simulink subsystem "Plant_Model_HT_Cooling_InnerLoop"  (R2022b)
settings: Solver=VariableStepAuto  StartTime=0.0  StopTime=10.0  RelTol=1e-3
values from neighbouring files (symbols this model uses):
  air_cp = 1004    [All_Properties.mat]    (also in cathode_subsystem_parameters.m; thermal_subsystem_parameters.m)
  air_HC_min = 10    [All_Properties.mat]    (also in cathode_subsystem_parameters.m; thermal_subsystem_parameters.m)
  air_HC_nom = 100    [All_Properties.mat]    (also in cathode_subsystem_parameters.m; thermal_subsystem_parameters.m)
  air_rho = 1.2    [All_Properties.mat]    (also in cathode_subsystem_parameters.m; thermal_subsystem_parameters.m)
  air_vel_nom = 1    [All_Properties.mat]    (also in cathode_subsystem_parameters.m; thermal_subsystem_parameters.m)
  coolant_initial_pressure = 0.111325    [All_Properties.mat]    (also in cathode_subsystem_parameters.m; thermal_subsystem_parameters.m)
  coolant_initial_temperature = 313.15    [All_Properties.mat]    (also in cathode_subsystem_parameters.m = 293.15; thermal_subsystem_parameters.m = 293.15)
  coolant_num_layers = 20    [All_Properties.mat]    (also in Plant_Model_HT_Cooling_Parameters.m; cathode_subsystem_parameters.m = 15; environment_parameters.m; stack_model_harness_parameters.m)
  coolant_num_passes = 12    [All_Properties.mat]    (also in Plant_Model_HT_Cooling_Parameters.m; cathode_subsystem_parameters.m = 20; environment_parameters.m; stack_model_harness_parameters.m)
  coolant_tube_D = 0.05    [All_Properties.mat]    (also in Plant_Model_HT_Cooling_Parameters.m; cathode_subsystem_parameters.m; environment_parameters.m; stack_model_harness_parameters.m)
  coolant_w_channels = 1    [All_Properties.mat]    (also in Plant_Model_HT_Cooling_Parameters.m; cathode_subsystem_parameters.m; environment_parameters.m; stack_model_harness_parameters.m)
  radiator_area_air = 0.1026    [All_Properties.mat]    (also in cathode_subsystem_parameters.m; thermal_subsystem_parameters.m)
  radiator_area_fins = 2.543625    [All_Properties.mat]    (also in cathode_subsystem_parameters.m; thermal_subsystem_parameters.m)
  radiator_area_primary = 0.444525    [All_Properties.mat]    (also in cathode_subsystem_parameters.m; thermal_subsystem_parameters.m = 2 * radiator_tube_length * radiator_width * (radiator_fin_ro)
  radiator_n_tubes = 20    [All_Properties.mat]    (also in cathode_subsystem_parameters.m; thermal_subsystem_parameters.m)
  radiator_tube_height = 0.0015    [All_Properties.mat]    (also in cathode_subsystem_parameters.m; thermal_subsystem_parameters.m)
  radiator_tube_length = 0.45    [All_Properties.mat]    (also in cathode_subsystem_parameters.m; thermal_subsystem_parameters.m)
  radiator_width = 0.025    [All_Properties.mat]    (also in cathode_subsystem_parameters.m; thermal_subsystem_parameters.m)
  stack_area = 300    [All_Properties.mat]    (also in Plant_Model_HT_Cooling_Parameters.m = 280; cathode_subsystem_parameters.m = 280; stack_model_parameters.m = 280; stack_subsystem_parameters.m)
  tcp_time_constant = 2    [All_Properties.mat]    (also in Plant_Model_HT_Cooling_Parameters.m; cathode_subsystem_parameters.m; thermal_subsystem_parameters.m)
  tcv_orifice_diameter = 0.045    [All_Properties.mat]    (also in Plant_Model_HT_Cooling_Parameters.m; cathode_subsystem_parameters.m; thermal_subsystem_parameters.m)
  tcv_time_constant = 0.2    [All_Properties.mat]    (also in Plant_Model_HT_Cooling_Parameters.m; cathode_subsystem_parameters.m; thermal_subsystem_parameters.m)
libraries: fl_lib x50, nesl_utility x40, SimscapeFluids_lib x7, eeGeneralControl x1
settings Model: Creator=stefan.notter  LastModifiedBy=stefan.notter

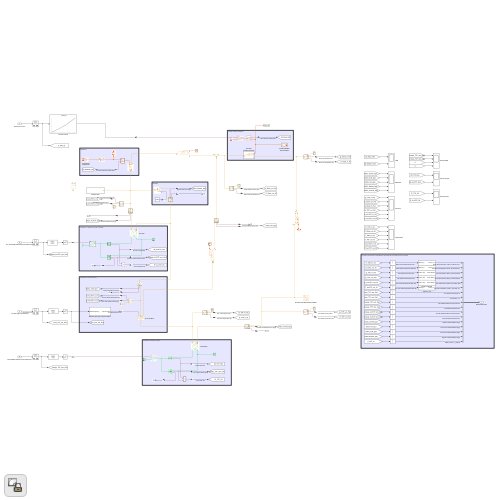
[thumbnail: Simulink's stored preview of the top-level diagram]
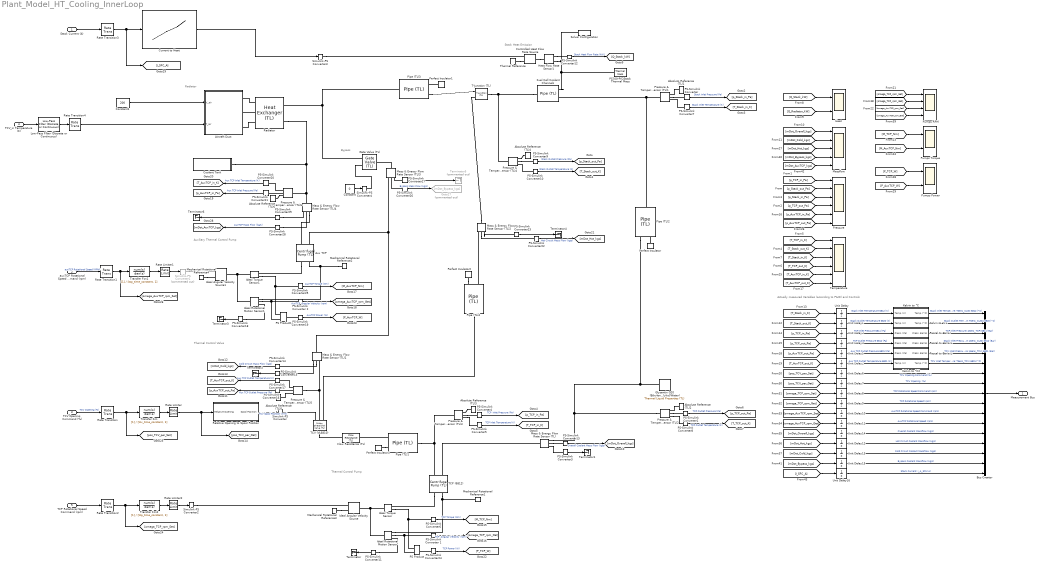
== system Plant_Model_HT_Cooling_InnerLoop ==
  note: Bypass
  note: Thermal Control Valve
  note: Actually measured Variables (according to P&ID) and Controls
  note: Stack Heat Emission
  note: Thermal Control Pump
  note: Radiator
  note: Auxiliary Thermal Control Pump
  Stack Current (A) : Inport
  auxTCP Rotational Speed Command (rpm) : Inport  Port=2
  TCV Opening Command (%) : Inport  Port=3
  TCV_in Temperature (K) : Inport  Port=4
  TCP Rotational Speed Command (rpm) : Inport  Port=5
  Absolute Reference (TL){1..6} (6 alike) : fl_lib/Thermal Liquid/Elements/Absolute Reference (TL)
  Aircraft Duct : Subsystem
  Aux TCP : SimscapeFluids_lib/Thermal Liquid/Pumps & Motors/Centrifugal Pump (TL)  pump_parameterization=fluids.thermal_liquid.pumps_motors.enum.CentrifugalPumpParameterization.Nominal  capacity_ref_nominal=6000/60 lpm  head_ref_nominal=|  power_ref_nominal=0.3 kW  head_ref_max=|  capacity_ref_max=12000/60 lpm  omega_ref_analytic=3500 rpm  flow_rate_1D_TLU=[1000, 2000, 3000, 4000, 5000, 6000, 7000, 8000, 9000, 1000] lpm  head_1D_TLU=[50, 47.5, 45, 40, 35, 25] m  power_1D_TLU=[.6, .75, .85, .93, .98, .99] kW  omega_ref_1D=3500 rpm  rho_ref_1D=998.21 kg/m^3  flow_rate_2D_TLU=[16.67, 23.33, 30, 40, 53.33, 60] lpm  omega_2D_TLU=[2450, 2800, 3150, 3500] rpm  head_2D_TLU=[25, 32.7, 42.5, 50; 24, 31.7, 41, 49; 22.7, 30.5, 39, 47.5; 20, 28, 36, 45; 15.7, 24, 32, 40; 12.5, 21, 29.5, 37.5] m  power_2D_TLU=[.28, .38, .5, .6; .31, .41, .55, .68; .33, .44, .6, .75; .36, .48, .65, .83; .38, .53, .72, .93; .39, .55, .75, .97] kW  rho_ref_2D=998.21 kg/m^3  diameter_ratio=1  mech_orientation=fluids.thermal_liquid.pumps_motors.enum.CentrifugalPumpMechOrientation.Positive  area=9.6211275016187417927918453612935e-4 m^2
      head_ref_nominal=|
      | 1.2*10^5/(1000*9.81)
      |  m
      head_ref_max=|
      | 1.55*10^5/(1000*9.81)
      |  m
      settings: InternalSimscapePortConfiguration="{\"Bottom\":[],\"Left\":[{\"id\":\"A\",\"label\":\"A\",\"type\":\"foundation.thermal_liquid.thermal_liquid\"},{\"id\":\"B\",\"label\":\"B\",\"type\":\"foundation.thermal_liquid.thermal_liquid\"}],\"Right\":[{\"id\":\"R\",\"label\":\"R\",\"type\":\"foundation.mechanical.rotational.rotational\"},{\"id\":\"C\",\"label\":\"C\",\"type\":\"foundation.mechanical.rotational.rotational\"}],\"Top\":[]}"
  Bus Creator : BusCreator  Inputs=17
  Constant : Constant  Value=0
  Constant1 : Constant  Value=200
  Controlled Heat Flow Rate Source : fl_lib/Thermal/Thermal Sources/Controlled Heat Flow Rate Source
  Coolant Tank : Subsystem  Tag=PublishSubsystem  mask(Coolant Tank){A=0.1, x_init=0.08}
      mask prompts: A "Tank area (m^2)"; x_init "Initial coolant level (m)"
      mask help: This subsystem models an expansion tank for the coolant system.
  Current to Heat : Lookup_n-D  NumberOfTableDimensions=1  BreakpointsForDimension1=[0:50:400]  Table=[0, 9932, 21438, 33442,47123, 59491, 77033, 93585, 112042]  InternalRulePriority=Speed  RndMeth=Simplest
  Flow Resistance (TL) : fl_lib/Thermal Liquid/Elements/Flow Resistance (TL)  delta_p_nominal=0.05 bar  mdot_nominal=1 kg/s  area=pi*tcv_orifice_diameter^2/4 m^2  laminar_fraction=1e-3
  Fuel Cell Coolant Channels : fl_lib/Thermal Liquid/Elements/Pipe (TL)  length=sqrt(stack_area) * coolant_num_passes cm  area=coolant_w_channels^2 * coolant_num_layers cm^2  Dh=coolant_w_channels cm  length_add=10 cm  roughness=15e-5 m  Re_lam=2000  Re_tur=4000  shape_factor=64  Nu_lam=3.66  dynamic_compressibility=simscape.enum.onoff.on  inertia=simscape.enum.onoff.off  p0=coolant_initial_pressure MPa  T0=coolant_initial_temperature K  mdot0=0 kg/s
  Gate Valve (TL) : SimscapeFluids_lib/Thermal Liquid/Valves & Orifices/Flow Control Valves/Gate Valve (TL)  diam_orifice=0.01 m  S_min=0 m  area_leak=1e-12 m^2  smoothing_factor=0.01  area=0.01 m^2  Cd=0.7  Re_c=12
      settings: InternalSimscapePortConfiguration="{\"Bottom\":[],\"Left\":[{\"id\":\"A\",\"label\":\"A\",\"type\":\"foundation.thermal_liquid.thermal_liquid\"},{\"id\":\"S\",\"label\":\"S\",\"type\":\"input\"}],\"Right\":[{\"id\":\"B\",\"label\":\"B\",\"type\":\"foundation.thermal_liquid.thermal_liquid\"}],\"Top\":[]}"
  Glysantin G20 (Ethylenglykol/Water) : SimscapeFluids_lib/Thermal Liquid/Utilities/Thermal Liquid Properties (TL)  fluid_list=fluids.thermal_liquid.utilities.enum.thermal_liquid_fluid_list.ethylene_glycol  concentration_param_EG=fluids.thermal_liquid.utilities.enum.thermal_liquid_concentration.volume_fraction  concentration_param_PG=fluids.thermal_liquid.utilities.enum.thermal_liquid_concentration.volume_fraction  c_mass_SW=3.5e-3  c_mass_EG=0.1  c_mass_PG=0.1  c_mass_GL=0.1  c_vol_EG=0.5  c_vol_PG=0.1  beta_const_EG=2.1791 GPa  beta_const_PG=2.1791 GPa  beta_const_GL=2.1791 GPa  p_min_EG=0.01 MPa  p_min_PG=0.01 MPa  p_min_GL=0.01 MPa  p_max_EG=50 MPa  p_max_PG=50 MPa  p_max_GL=50 MPa  p_atm=coolant_initial_pressure MPa
  Goto27 : Goto  Commented=on  GotoTag=mDot_Bypass_kgs
  Heat : Scope  NumInputPorts=2
  Heat Flow Rate Sensor1 : fl_lib/Thermal/Thermal Sensors/Heat Flow Rate Sensor
  Ideal Angular Velocity Source : fl_lib/Mechanical/Mechanical Sources/Ideal Angular Velocity Source
  Ideal Angular Velocity Source1 : fl_lib/Mechanical/Mechanical Sources/Ideal Angular Velocity Source
  Ideal Rotational Motion Sensor : fl_lib/Mechanical/Mechanical Sensors/Ideal Rotational Motion Sensor  reference=foundation.enum.MeasurementReference.difference  acceleration_port=false  velocity_port=true  position_port=true  wrap_angle=false  offset=0 rad
  Ideal Rotational Motion Sensor1 : fl_lib/Mechanical/Mechanical Sensors/Ideal Rotational Motion Sensor  reference=foundation.enum.MeasurementReference.difference  acceleration_port=false  velocity_port=true  position_port=true  wrap_angle=false  offset=0 rad
  Ideal Torque Sensor : fl_lib/Mechanical/Mechanical Sensors/Ideal Torque Sensor
  Ideal Torque Sensor1 : fl_lib/Mechanical/Mechanical Sensors/Ideal Torque Sensor
  Kelvin to °C : Subsystem
  Kelvin to °C1 : Subsystem
  Kelvin to °C2 : Subsystem
  Low-Pass Filter (Discrete or Continuous) : eeGeneralControl/Low-Pass Filter (Discrete or Continuous)  K=1  T=1  B=inf  A=-inf  init_option=Inherited from block input  x0=0  Ts=-1
  Mass & Energy Flow Rate Sensor (TL){,1..4} (5 alike) : fl_lib/Thermal Liquid/Sensors/Mass & Energy Flow Rate Sensor (TL)
      settings: InternalSimscapePortConfiguration="{\"Bottom\":[],\"Left\":[{\"id\":\"A\",\"label\":\"A\",\"type\":\"foundation.thermal_liquid.thermal_liquid\"}],\"Right\":[{\"id\":\"B\",\"label\":\"B\",\"type\":\"foundation.thermal_liquid.thermal_liquid\"},{\"id\":\"M\",\"label\":\"M\",\"type\":\"output\"},{\"id\":\"PHI\",\"label\":\"Phi\",\"type\":\"output\"}],\"Top\":[]}"
  Massflow : Scope  NumInputPorts=5
  Mechanical Rotational Reference{1..4} (4 alike) : fl_lib/Mechanical/Rotational Elements/Mechanical Rotational Reference
  PS Product : fl_lib/Physical Signals/Functions/PS Product
  PS Product1 : fl_lib/Physical Signals/Functions/PS Product
  PS-Simulink Converter{,1,3..5,7..11,13..18,20..23,26..29} (24 alike) : nesl_utility/PS-Simulink Converter  PhysicalDomain=network_engine_domain  SubClassName=ps_output  LeftPortType=input  RightPortType=output  PseudoPeriodic=off  Frequencies=[]  VectorFormat=inherit  Unit=inherit  AffineConversion=off
  PS-Simulink Converter 1 : nesl_utility/PS-Simulink Converter  PhysicalDomain=network_engine_domain  SubClassName=ps_output  LeftPortType=input  RightPortType=output  PseudoPeriodic=off  Frequencies=[]  VectorFormat=1-D array  Unit=rpm  AffineConversion=off
  PS-Simulink Converter 2 : nesl_utility/PS-Simulink Converter  PhysicalDomain=network_engine_domain  SubClassName=ps_output  LeftPortType=input  RightPortType=output  PseudoPeriodic=off  Frequencies=[]  VectorFormat=1-D array  Unit=rpm  AffineConversion=off
  PS-Simulink Converter12 : nesl_utility/PS-Simulink Converter  PhysicalDomain=network_engine_domain  SubClassName=ps_output  LeftPortType=input  RightPortType=output  PseudoPeriodic=off  Frequencies=[]  VectorFormat=1-D array  Unit=kW  AffineConversion=off
  PS-Simulink Converter19 : nesl_utility/PS-Simulink Converter  PhysicalDomain=network_engine_domain  SubClassName=ps_output  LeftPortType=input  RightPortType=output  PseudoPeriodic=off  Frequencies=[]  VectorFormat=inherit  Unit=W  AffineConversion=off
  PS-Simulink Converter24 : nesl_utility/PS-Simulink Converter  PhysicalDomain=network_engine_domain  SubClassName=ps_output  LeftPortType=input  RightPortType=output  PseudoPeriodic=off  Frequencies=[]  VectorFormat=inherit  Unit=W  AffineConversion=off
  PS-Simulink Converter25 : nesl_utility/PS-Simulink Converter  PhysicalDomain=network_engine_domain  SubClassName=ps_output  LeftPortType=input  RightPortType=output  PseudoPeriodic=off  Frequencies=[]  VectorFormat=inherit  Unit=N*m  AffineConversion=off
  PS-Simulink Converter6 : nesl_utility/PS-Simulink Converter  PhysicalDomain=network_engine_domain  SubClassName=ps_output  LeftPortType=input  RightPortType=output  PseudoPeriodic=off  Frequencies=[]  VectorFormat=inherit  Unit=N*m  AffineConversion=off
  PS100-P02Stack Thermal Mass : fl_lib/Thermal/Thermal Elements/Thermal Mass  mass=stack_thermal_mass kg  sp_heat=stack_specific_heat J/kg/K  num_ports=foundation.enum.numPorts2.one  T_specify=on  T_priority=High  T=coolant_initial_temperature K  T_nominal_specify=off  T_nominal_unit=K  T_nominal_value=1  Q_specify=off  Q_priority=None  Q=20e3 W  Q_nominal_specify=off  Q_nominal_unit=W  Q_nominal_value=1
  Pascal to Bar(a) : Subsystem
  Pascal to Bar(a)1 : Subsystem
  Pascal to Bar(a)2 : Subsystem
  Perfect Insulator{,1..3} (4 alike) : fl_lib/Thermal/Thermal Elements/Perfect Insulator  T_specify=off  T_priority=None  T=293.15 K  T_nominal_specify=off  T_nominal_unit=K  T_nominal_value=1
  Pipe (TL)1 : fl_lib/Thermal Liquid/Elements/Pipe (TL)  length=0.5 m  area=pi*coolant_tube_D^2/4 m^2  Dh=pi*coolant_tube_D*0.9 m  length_add=0.5 m  roughness=15e-6 m  Re_lam=2000  Re_tur=4000  shape_factor=64  Nu_lam=3.66  dynamic_compressibility=simscape.enum.onoff.on  inertia=simscape.enum.onoff.off  p0=coolant_initial_pressure MPa  T0=coolant_initial_temperature K  mdot0=0 kg/s
  Pipe (TL)2 : fl_lib/Thermal Liquid/Elements/Pipe (TL)  length=0.5 m  area=pi*coolant_tube_D^2/4 m^2  Dh=pi*coolant_tube_D*0.9 m  length_add=1 m  roughness=15e-6 m  Re_lam=2000  Re_tur=4000  shape_factor=64  Nu_lam=3.66  dynamic_compressibility=simscape.enum.onoff.on  inertia=simscape.enum.onoff.off  p0=coolant_initial_pressure MPa  T0=coolant_initial_temperature K  mdot0=0 kg/s
  Pipe (TL)3 : fl_lib/Thermal Liquid/Elements/Pipe (TL)  length=1 m  area=pi*coolant_tube_D^2/4 m^2  Dh=pi*coolant_tube_D*0.9 m  length_add=1 m  roughness=15e-6 m  Re_lam=2000  Re_tur=4000  shape_factor=64  Nu_lam=3.66  dynamic_compressibility=simscape.enum.onoff.on  inertia=simscape.enum.onoff.off  p0=coolant_initial_pressure MPa  T0=coolant_initial_temperature K  mdot0=0 kg/s
  Pipe (TL)4 : fl_lib/Thermal Liquid/Elements/Pipe (TL)  length=0.5 m  area=pi*coolant_tube_D^2/4 m^2  Dh=pi*coolant_tube_D*0.9 m  length_add=1 m  roughness=15e-6 m  Re_lam=2000  Re_tur=4000  shape_factor=64  Nu_lam=3.66  dynamic_compressibility=simscape.enum.onoff.on  inertia=simscape.enum.onoff.off  p0=coolant_initial_pressure MPa  T0=coolant_initial_temperature K  mdot0=0 kg/s
  Pressure : Scope  NumInputPorts=6
  Pressure & Temperature Sensor (TL){1..6} (6 alike) : fl_lib/Thermal Liquid/Sensors/Pressure & Temperature Sensor (TL)
      settings: InternalSimscapePortConfiguration="{\"Bottom\":[],\"Left\":[{\"id\":\"A\",\"label\":\"A\",\"type\":\"foundation.thermal_liquid.thermal_liquid\"}],\"Right\":[{\"id\":\"B\",\"label\":\"B\",\"type\":\"foundation.thermal_liquid.thermal_liquid\"},{\"id\":\"P\",\"label\":\"P\",\"type\":\"output\"},{\"id\":\"T\",\"label\":\"T\",\"type\":\"output\"}],\"Top\":[]}"
  Pumps Power : Scope  NumInputPorts=2
  Pumps RPM : Scope  NumInputPorts=4
  Pumps Torque : Scope  NumInputPorts=2
  Radiator : SimscapeFluids_lib/Fluid Network Interfaces/Heat Exchangers/Heat Exchanger (TL)  hex_type=3  shell_num=1  cross_type=4  NTU_TLU=[0.5, 1.0, 2.0, 3.0, 4.0, 5.0]  CR_TLU=[0.0, 0.25, 0.5, 0.75, 1.0]  eff_TLU=[0.3, 0.3, 0.3, 0.3, 0.3; 0.6, 0.55, 0.5, 0.47, 0.43; 0.85, 0.76, 0.68, 0.61, 0.55; 0.94, 0.83, 0.72, 0.65, 0.58; 0.98, 0.86, 0.75, 0.66, 0.58; 0.99, 0.86, 0.75, 0.66, 0.58]  R_wall=0.014/(381*radiator_n_tubes*radiator_width*radiator_tube_length) K/W  min_flow_area_1=radiator_n_tubes*(radiator_width*radiator_tube_height) m^2  Dh_press_1=4*(radiator_width*radiator_tube_height)/(2 * (radiator_width+radiator_tube_height)) m  liquid_volume_1=radiator_n_tubes*(radiator_width*radiator_tube_height)*radiator_tube_length m^3  Re_lam_1=2000  Re_tur_1=4000  pressure_loss_spec_1=2  pressure_loss_coeff_1=15  length_press_1=radiator_tube_length m  length_add_1=0.1 m  roughness_1=15e-6 m  Re_friction_TLU_1=[400.0, 1000.0, 1500.0, 3000.0, 4000.0, 6000.0, 10000.0, 20000.0, 40000.0, 60000.0, 100000.0, 100000000.0]  friction_factor_TLU_1=[0.264, 0.112, 0.071, 0.0417, 0.0387, 0.0268, 0.025, 0.0232, 0.0226, 0.022, 0.0214, 0.0214]  shape_factor_1=64  Re_Euler_TLU_1=[50.0, 500.0, 1000.0, 2000.0]  Euler_TLU_1=[4.4505, 0.6864, 0.4791, 0.3755]  heat_transfer_spec_1=2  heat_transfer_area_1=radiator_n_tubes*2*(radiator_tube_length*radiator_width+radiator_tube_length*radiator_tube_height) m^2  heat_coeff_1=2000 W/(m^2 * K)  length_heat_1=radiator_tube_length cm  Nu_lam_1=3.66  Re_Colburn_TLU_1=[100.0, 150.0, 1000.0]  Colburn_factor_TLU_1=[0.019, 0.013, 0.002]  Re_Nu_TLU_1=[100.0, 150.0, 1000.0]  Pr_Nu_TLU_1=[1.0, 10.0]  Nu_TLU_1=[3.72, 4.21; 3.75, 4.44; 4.21, 7.15]  fouling_factor_1=0 m^2*K/W  min_heat_coeff_1=5 W/(m^2 * K)  heat_transfer_area_2=radiator_area_primary+radiator_area_fins m^2  fouling_factor_2=0 m^2*K/W  min_heat_coeff_2=0.01 W/(m^2 * K)  dynamic_compressibility_1=1  T0_1=coolant_initial_temperature K  p0_1=coolant_initial_pressure MPa  mdot1_TLU=[.1, .2] kg/s  mdot2_TLU=[.2, .3] kg/s  SD_TLU=[35, 35; 50, 50] kW/K  Q_check=1  mdot_dp_TLU_1=[.1, .2] kg/s  p_diff_TLU_1=[.003, .005] MPa  T_ref_in_1=293.15 K  p_ref_in_1=0.101325 MPa  mdot_threshold_1=1e-3 kg/s  area_1=0.01 m^2
      settings: InternalSimscapePortConfiguration="{\"Bottom\":[],\"Left\":[{\"id\":\"A1\",\"label\":\"A1\",\"type\":\"foundation.thermal_liquid.thermal_liquid\"},{\"id\":\"B1\",\"label\":\"B1\",\"type\":\"foundation.thermal_liquid.thermal_liquid\"}],\"Right\":[{\"id\":\"H2\",\"label\":\"H2\",\"type\":\"foundation.thermal.thermal\"},{\"id\":\"C2\",\"label\":\"C2\",\"type\":\"input\"},{\"id\":\"HC2\",\"label\":\"HC2\",\"type\":\"input\"}],\"Top\":[]}"
  Rate Limiter : RateLimiter  RisingSlewLimit=45  FallingSlewLimit=-45  SampleTimeMode=inherited
  Rate Limiter1 : RateLimiter  RisingSlewLimit=1000  FallingSlewLimit=-1000  SampleTimeMode=inherited
  Rate Limiter2 : RateLimiter  RisingSlewLimit=1000  FallingSlewLimit=-1000  SampleTimeMode=inherited
  Rate Transition{,1..3} (4 alike) : RateTransition
  Rate Transition4 : RateTransition  InitialCondition=coolant_initial_temperature
  Relative Opening to Spool Position : Subsystem
  Simulink-PS Converter : nesl_utility/Simulink-PS Converter  PhysicalDomain=network_engine_domain  SubClassName=ps_input  LeftPortType=input  RightPortType=output  PseudoPeriodic=off  Frequencies=[]  NoiseDistribution=none  NoiseParameters=[]  Unit=mm  AffineConversion=off  FilteringAndDerivatives=provide  SimscapeFilterOrder=1  InputFilterTimeConstant=0.001  UdotUserProvided=0
  Simulink-PS Converter1 : nesl_utility/Simulink-PS Converter  Commented=on  PhysicalDomain=network_engine_domain  SubClassName=ps_input  LeftPortType=input  RightPortType=output  PseudoPeriodic=off  Frequencies=[]  NoiseDistribution=none  NoiseParameters=[]  Unit=rpm  AffineConversion=off  FilteringAndDerivatives=provide  SimscapeFilterOrder=1  InputFilterTimeConstant=0.001  UdotUserProvided=0
  Simulink-PS Converter2 : nesl_utility/Simulink-PS Converter  PhysicalDomain=network_engine_domain  SubClassName=ps_input  LeftPortType=input  RightPortType=output  PseudoPeriodic=off  Frequencies=[]  NoiseDistribution=none  NoiseParameters=[]  Unit=rpm  AffineConversion=off  FilteringAndDerivatives=provide  SimscapeFilterOrder=1  InputFilterTimeConstant=0.001  UdotUserProvided=0
  Simulink-PS Converter3 : nesl_utility/Simulink-PS Converter  PhysicalDomain=network_engine_domain  SubClassName=ps_input  LeftPortType=input  RightPortType=output  PseudoPeriodic=off  Frequencies=[]  NoiseDistribution=none  NoiseParameters=[]  Unit=J/s  AffineConversion=off  FilteringAndDerivatives=provide  SimscapeFilterOrder=1  InputFilterTimeConstant=0.001  UdotUserProvided=0
  Simulink-PS Converter4 : nesl_utility/Simulink-PS Converter  PhysicalDomain=network_engine_domain  SubClassName=ps_input  LeftPortType=input  RightPortType=output  PseudoPeriodic=off  Frequencies=[]  NoiseDistribution=none  NoiseParameters=[]  Unit=1  AffineConversion=off  FilteringAndDerivatives=provide  SimscapeFilterOrder=1  InputFilterTimeConstant=0.001  UdotUserProvided=0
  Solver Configuration : nesl_utility/Solver Configuration  PhysicalDomain=network_engine_domain  SubClassName=solver  LeftPortType=input  RightPortType=generic  Tones=[]  Harmonics=[]  SimulateNoise=off  Profile=off  UseLocalSampling=off  EnableSwitchedLinearOptims=on  FrequencyDomain=off  UseCCode=off  RelTol=0.001  AbsTol=1e-06  MinStep=1e-09  ToWorkspace=off  RevertToSquareIcSolve=off  NumHomotopyIterations=100  PhasorMode=off  PhasorModeNumHarmonics=1  ConsistencySolver=NEWTON_XTOL_AFTER_FTOL  IndexReductionMethod=DerivativeReplacement  DoDC=off  ResidualTolerance=1e-09  ConsistencyTolSource=GLOBAL  ConsistencyAbsTol=0.001  ConsistencyRelTol=0.001  ConsistencyTolFactor=0.001  UseLocalSolver=on  LocalSolverChoice=NE_BACKWARD_EULER_ADVANCER  ResolveIndetEquations=on  FunctionEvalNumThread=1  LocalSolverSampleTime=0.001  DoFixedCost=on  MaxNonlinIter=3  MaxModeIter=2  ComputeImpulses=off  ImpulseIterations=2  LinearAlgebra=auto  LinearAlgebraNumThread=0  EquationFormulation=NE_TIME_EF  DelaysMemoryBudget=1024  AutomaticFiltering=off  FilteringTimeConstant=0.001  PartitionStorageMethod=AS_NEEDED  PartitionMemoryBudget=1024  PartitionMethod=ROBUST
  T-Junction (TL) : SimscapeFluids_lib/Thermal Liquid/Pipes & Fittings/T-Junction (TL)  area_main=pi*coolant_tube_D^2/4 m^2  area_branch=pi*coolant_tube_D^2/4 m^2  junction_spec=fluids.thermal_liquid.pipes_fittings.enum.ThreeWayJunctionSpec.Standard  k_main_converge=1.12  k_main_diverge=1.12  k_branch_converge=1.12  k_branch_diverge=1.12  Re_c=150  mdot_A_specify=off  mdot_A_priority=High  mdot_A=0 kg/s  mdot_A_nominal_specify=off  mdot_A_nominal_unit=kg/s  mdot_A_nominal_value=1  mdot_B_specify=off  mdot_B_priority=High  mdot_B=0 kg/s  mdot_B_nominal_specify=off  mdot_B_nominal_unit=kg/s  mdot_B_nominal_value=1  mdot_C_specify=off  mdot_C_priority=High  mdot_C=0 kg/s  mdot_C_nominal_specify=off  mdot_C_nominal_unit=kg/s  mdot_C_nominal_value=1  Phi_A_specify=off  Phi_A_priority=None  Phi_A=0 kW  Phi_A_nominal_specify=off  Phi_A_nominal_unit=kW  Phi_A_nominal_value=1  Phi_B_specify=off  Phi_B_priority=None  Phi_B=0 kW  Phi_B_nominal_specify=off  Phi_B_nominal_unit=kW  Phi_B_nominal_value=1  Phi_C_specify=off  Phi_C_priority=None  Phi_C=0 kW  Phi_C_nominal_specify=off  Phi_C_nominal_unit=kW  Phi_C_nominal_value=1
      settings: InternalSimscapePortConfiguration="{\"Bottom\":[{\"id\":\"C\",\"label\":\"C\",\"type\":\"foundation.thermal_liquid.thermal_liquid\"}],\"Left\":[{\"id\":\"A\",\"label\":\"A\",\"type\":\"foundation.thermal_liquid.thermal_liquid\"}],\"Right\":[{\"id\":\"B\",\"label\":\"B\",\"type\":\"foundation.thermal_liquid.thermal_liquid\"}],\"Top\":[]}"
  TCP (6812) : SimscapeFluids_lib/Thermal Liquid/Pumps & Motors/Centrifugal Pump (TL)  pump_parameterization=fluids.thermal_liquid.pumps_motors.enum.CentrifugalPumpParameterization.Nominal  capacity_ref_nominal=6000/60 lpm  head_ref_nominal=|  power_ref_nominal=0.3 kW  head_ref_max=|  capacity_ref_max=12000/60 lpm  omega_ref_analytic=3500 rpm  flow_rate_1D_TLU=[1000, 2000, 3000, 4000, 5000, 6000, 7000, 8000, 9000, 1000] lpm  head_1D_TLU=[50, 47.5, 45, 40, 35, 25] m  power_1D_TLU=[.6, .75, .85, .93, .98, .99] kW  omega_ref_1D=3500 rpm  rho_ref_1D=998.21 kg/m^3  flow_rate_2D_TLU=[16.67, 23.33, 30, 40, 53.33, 60] lpm  omega_2D_TLU=[2450, 2800, 3150, 3500] rpm  head_2D_TLU=[25, 32.7, 42.5, 50; 24, 31.7, 41, 49; 22.7, 30.5, 39, 47.5; 20, 28, 36, 45; 15.7, 24, 32, 40; 12.5, 21, 29.5, 37.5] m  power_2D_TLU=[.28, .38, .5, .6; .31, .41, .55, .68; .33, .44, .6, .75; .36, .48, .65, .83; .38, .53, .72, .93; .39, .55, .75, .97] kW  rho_ref_2D=998.21 kg/m^3  diameter_ratio=1  mech_orientation=fluids.thermal_liquid.pumps_motors.enum.CentrifugalPumpMechOrientation.Positive  area=9.6211275016187417927918453612935e-4 m^2
      head_ref_nominal=|
      | 1.2*10^5/(1000*9.81)
      |  m
      head_ref_max=|
      | 1.55*10^5/(1000*9.81)
      |  m
      settings: InternalSimscapePortConfiguration="{\"Bottom\":[],\"Left\":[{\"id\":\"A\",\"label\":\"A\",\"type\":\"foundation.thermal_liquid.thermal_liquid\"},{\"id\":\"B\",\"label\":\"B\",\"type\":\"foundation.thermal_liquid.thermal_liquid\"}],\"Right\":[{\"id\":\"R\",\"label\":\"R\",\"type\":\"foundation.mechanical.rotational.rotational\"},{\"id\":\"C\",\"label\":\"C\",\"type\":\"foundation.mechanical.rotational.rotational\"}],\"Top\":[]}"
  TCV (VL6810) : SimscapeFluids_lib/Thermal Liquid/Valves & Orifices/Directional Control Valves/3-Way Directional Valve (TL)  open_orifices_pos=fluids.thermal_liquid.valves.directional_control_valves.enum.OpenOrifices3Way.PA  open_orifices_neg=fluids.thermal_liquid.valves.directional_control_valves.enum.OpenOrifices3Way.AT  area_spec=fluids.thermal_liquid.valves.directional_control_valves.enum.area_spec.identical  valve_spec=fluids.thermal_liquid.valves.directional_control_valves.enum.ValveSpec.Linear  del_S_max=5e-3 m  area_max=pi*tcv_orifice_diameter^2/4 m^2  del_S_TLU=[0, .002, .004, .007, .017] m  valve_area_TLU=[1e-09, 2.0352e-07, 4.0736e-05, .00011438, .00034356] m^2  del_S_flow_TLU=[0, .002, .004, .007, .017] m  p_diff_TLU=[.3, .5, .7] bar  vol_flow_TLU=1e-3 * [1.7e-05, 2e-05, 2.6e-05; .0035, .0045, .0053; .7, .9, 1.06; 1.96, 2.5, 3; 6, 7.7, 9.13] lpm  mdot_TLU=[1.7e-05, 2e-05, 2.6e-05; .0035, .0045, .0053; .7, .9, 1.06; 1.96, 2.5, 3; 6, 7.7, 9.13] kg/s  T_ref_in=293.15 K  p_ref_in=0.101325 MPa  area_leak=tcv_leakage_area m^2  Cd=0.7  Re_c=12  smoothing_factor=0.01  pressure_recovery=simscape.enum.onoff.off  area=pi*coolant_tube_D^2/4 m^2  S_max_PA=2.5e-3 m  del_S_max_PA=0.005 m  area_max_PA=1e-4 m^2  del_S_TLU_PA=[0, .002, .004, .007, .017] m  valve_area_TLU_PA=[1e-09, 2.0352e-07, 4.0736e-05, .00011438, .00034356] m^2  del_S_flow_TLU_PA=[0, .002, .004, .007, .017] m  p_diff_TLU_PA=[.3, .5, .7] MPa  vol_flow_TLU_PA=1e-3 * [1.7e-05, 2e-05, 2.6e-05; .0035, .0045, .0053; .7, .9, 1.06; 1.96, 2.5, 3; 6, 7.7, 9.13] m^3/s  mdot_TLU_PA=[1.7e-05, 2e-05, 2.6e-05; .0035, .0045, .0053; .7, .9, 1.06; 1.96, 2.5, 3; 6, 7.7, 9.13] kg/s  S_max_AT=-2.5e-3 m  del_S_max_AT=0.005 m  area_max_AT=1e-4 m^2  del_S_TLU_AT=[0, .002, .004, .007, .017] m  valve_area_TLU_AT=[1e-09, 2.0352e-07, 4.0736e-05, .00011438, .00034356] m^2  del_S_flow_TLU_AT=[0, .002, .004, .007, .017] m  p_diff_TLU_AT=[.3, .5, .7] MPa  vol_flow_TLU_AT=1e-3 * [1.7e-05, 2e-05, 2.6e-05; .0035, .0045, .0053; .7, .9, 1.06; 1.96, 2.5, 3; 6, 7.7, 9.13] m^3/s  mdot_TLU_AT=[1.7e-05, 2e-05, 2.6e-05; .0035, .0045, .0053; .7, .9, 1.06; 1.96, 2.5, 3; 6, 7.7, 9.13] kg/s  S_max_PT=2.5e-3 m  del_S_max_PT=0.005 m  area_max_PT=1e-4 m^2  del_S_TLU_PT=[0, .002, .004, .007, .017] m  valve_area_TLU_PT=[1e-09, 2.0352e-07, 4.0736e-05, .00011438, .00034356] m^2  del_S_flow_TLU_PT=[0, .002, .004, .007, .017] m  p_diff_TLU_PT=[.3, .5, .7] MPa  vol_flow_TLU_PT=1e-3 * [1.7e-05, 2e-05, 2.6e-05; .0035, .0045, .0053; .7, .9, 1.06; 1.96, 2.5, 3; 6, 7.7, 9.13] m^3/s  mdot_TLU_PT=[1.7e-05, 2e-05, 2.6e-05; .0035, .0045, .0053; .7, .9, 1.06; 1.96, 2.5, 3; 6, 7.7, 9.13] kg/s
      settings: InternalSimscapePortConfiguration="{\"Bottom\":[],\"Left\":[{\"id\":\"A\",\"label\":\"A\",\"type\":\"foundation.thermal_liquid.thermal_liquid\"}],\"Right\":[{\"id\":\"S\",\"label\":\"S\",\"type\":\"input\"},{\"id\":\"P\",\"label\":\"P\",\"type\":\"foundation.thermal_liquid.thermal_liquid\"},{\"id\":\"T\",\"label\":\"T\",\"type\":\"foundation.thermal_liquid.thermal_liquid\"}],\"Top\":[]}"
  Temperature : Scope  NumInputPorts=6
  Terminator{,1..4,6} (6 alike) : Terminator
  Terminator5 : Terminator  Commented=on
  Thermal Reference : fl_lib/Thermal/Thermal Elements/Thermal Reference
  Transfer Fcn : TransferFcn  Denominator=[tcv_time_constant, 1]  ContinuousStateAttributes='tcv_opening'
  Transfer Fcn1 : TransferFcn  Denominator=[tcp_time_constant, 1]  ContinuousStateAttributes='tcv_opening'
  Transfer Fcn2 : TransferFcn  Denominator=[tcp_time_constant, 1]  ContinuousStateAttributes='tcv_opening'
  Unit Delay : UnitDelay  InitialCondition=coolant_initial_temperature  SampleTime=-1  HasFrameUpgradeWarning=on
  Unit Delay1 : UnitDelay  InitialCondition=coolant_initial_temperature  SampleTime=-1  HasFrameUpgradeWarning=on
  Unit Delay{6..16} (11 alike) : UnitDelay  SampleTime=-1  HasFrameUpgradeWarning=on
  Unit Delay2 : UnitDelay  InitialCondition=coolant_initial_temperature  SampleTime=-1  HasFrameUpgradeWarning=on
  Unit Delay3 : UnitDelay  InitialCondition=coolant_initial_pressure  SampleTime=-1  HasFrameUpgradeWarning=on
  Unit Delay4 : UnitDelay  InitialCondition=coolant_initial_pressure  SampleTime=-1  HasFrameUpgradeWarning=on
  Unit Delay5 : UnitDelay  InitialCondition=coolant_initial_pressure  SampleTime=-1  HasFrameUpgradeWarning=on
  Measurement Bus : Outport
  wires:
  PS-Simulink Converter 1/1 -> [omega_TCP_rpm_Get]  "TCP  Angular Velocity (rpm)"
  Relative Opening to Spool Position/1(Spool Position) -> Simulink-PS Converter/1  "TCV Spool Position (mm)"
  PS-Simulink Converter11/1 -> Terminator/1
  PS-Simulink Converter6/1 -> [M_TCP_Nm]  "TCP Torque (Nm)"
  Bus Creator/1 -> Measurement Bus/1
  PS-Simulink Converter9/1 -> [p_Stack_out_Pa]  "Stack Outlet Pressure (Pa)"
  PS-Simulink Converter10/1 -> [T_Stack_out_K]  "Stack Outlet Temperature (K)"
  PS-Simulink Converter/1 -> [p_Stack_in_Pa]  "Stack Inlet Pressure (Pa)"
  PS-Simulink Converter7/1 -> [T_Stack_in_K]  "Stack Inlet Temperature (K)"
  PS-Simulink Converter5/1 -> [T_TCP_in_K]  "TCP Inlet Temperature (K)"
  PS-Simulink Converter4/1 -> [p_TCP_in_Pa]  "TCP  Inlet Pressure (Pa)"
  PS-Simulink Converter1/1 -> [p_TCP_out_Pa]  "TCP Outlet Pressure (Pa)"
  PS-Simulink Converter8/1 -> [T_TCP_out_K]  "TCP Outlet Temperature (K)"
  PS-Simulink Converter12/1 -> [Q_Stack_kW]  "Stack Heat Flow Rate (kW)"
  [p_TCP_out_Pa] -> Pressure/4
  [p_Stack_in_Pa] -> Pressure/3
  [p_Stack_out_Pa] -> Pressure/2
  [p_TCP_in_Pa] -> Pressure/1
  [T_Stack_in_K] -> Temperature/3
  [T_TCP_out_K] -> Temperature/4
  [T_TCP_in_K] -> Temperature/1
  [T_Stack_out_K] -> Temperature/2
  [Q_Stack_kW] -> Heat/1
  [Q_Radiator_kW] -> Heat/2
  PS-Simulink Converter3/1 -> Terminator1/1
  PS-Simulink Converter13/1 -> [mDot_Overall_kgs]  "Overall Coolant Mass Flow (kg/s)"
  PS-Simulink Converter15/1 -> Terminator2/1
  PS-Simulink Converter14/1 -> [mDot_Cold_kgs]  "Cold Circuit Mass Flow (kg/s)"
  [mDot_Overall_kgs] -> Massflow/1
  [mDot_Cold_kgs] -> Massflow/2
  [T_Stack_out_K] -> Unit Delay1/1
  [T_Stack_in_K] -> Unit Delay/1
  [p_TCP_in_Pa] -> Unit Delay3/1
  [p_TCP_out_Pa] -> Unit Delay4/1
  PS-Simulink Converter16/1 -> [p_AuxTCP_out_Pa]  "Aux TCP Outlet Pressure (Pa)"
  PS-Simulink Converter17/1 -> [T_AuxTCP_out_K]  "Aux TCP Outlet Temperature (K)"
  [p_AuxTCP_in_Pa] -> Pressure/5
  [T_AuxTCP_out_K] -> Temperature/6
  [p_AuxTCP_out_Pa] -> Unit Delay5/1
  [T_AuxTCP_out_K] -> Unit Delay2/1
  [pos_TCV_per_Set] -> Unit Delay6/1
  [omega_TCP_rpm_Set] -> Pumps RPM/1
  [M_TCP_Nm] -> Pumps Torque/1
  [M_AuxTCP_Nm] -> Pumps Torque/2
  PS-Simulink Converter21/1 -> [p_AuxTCP_in_Pa]  "Aux TCP Inlet Pressure (Pa)"
  PS-Simulink Converter20/1 -> [T_AuxTCP_in_K]  "Aux TCP Inlet Temperature (K)"
  [T_AuxTCP_in_K] -> Temperature/5
  [p_AuxTCP_out_Pa] -> Pressure/6
  PS-Simulink Converter22/1 -> [mDot_Hot_kgs]  "Hot Circuit Mass Flow (kg/s)"
  PS-Simulink Converter23/1 -> Terminator4/1
  [mDot_Hot_kgs] -> Massflow/3
  TCP Rotational Speed Command (rpm)/1 -> Rate Transition2/1
  PS-Simulink Converter24/1 -> [P_TCP_W]  "TCP Power (W)"
  [P_TCP_W] -> Pumps Power/1
  PS-Simulink Converter18/1 -> Terminator3/1
  PS-Simulink Converter 2/1 -> [omega_AuxTCP_rpm_Get]  "AuxTCP  Angular Velocity (rpm)"
  PS-Simulink Converter25/1 -> [M_AuxTCP_Nm]  "AuxTCP Torque (Nm)"
  PS-Simulink Converter19/1 -> [P_AuxTCP_W]  "AuxTCP Power (W)"
  [P_AuxTCP_W] -> Pumps Power/2
  Unit Delay/1 -> Kelvin to °C/1(Temp. (K))  "Stack Inlet Temperature 6812 (K)"
  Unit Delay1/1 -> Kelvin to °C1/1(Temp. (K))  "Stack Outlet Temperature 6820 (K)"
  Unit Delay2/1 -> Kelvin to °C2/1(Temp. (K))  "Aux TCP Outlet Temperature 6801 (K)"
  Unit Delay3/1 -> Pascal to Bar(a)/1(Press. (Pa))  "TCP Inlet Pressure 6811 (Pa)"
  Unit Delay4/1 -> Pascal to Bar(a)1/1(Press. (Pa))  "TCP Outlet Pressure 6812 (Pa)"
  Unit Delay5/1 -> Pascal to Bar(a)2/1(Press. (Pa))  "Aux TCP Outlet Pressure 6801 (Pa)"
  Unit Delay6/1 -> Bus Creator/7  "TCV Opening Command (%)"
  Rate Limiter/1 -> Relative Opening to Spool Position/1(Relative Opening), [pos_TCV_per_Get]
  Rate Limiter1/1 -> Simulink-PS Converter1/1
  Rate Limiter2/1 -> Simulink-PS Converter2/1
  TCV Opening Command (%)/1 -> Rate Transition/1  "TCV Opening (%)"
  auxTCP Rotational Speed Command (rpm)/1 -> Rate Transition1/1  "auxTCP Rotational Speed (RPM)"
  [pos_TCV_per_Get] -> Unit Delay7/1
  Unit Delay7/1 -> Bus Creator/8  "TCV Opening  (%)"
  Unit Delay9/1 -> Bus Creator/10  "TCP Rotational Speed (rpm)"
  [omega_TCP_rpm_Get] -> Unit Delay9/1
  [omega_TCP_rpm_Set] -> Unit Delay8/1
  Unit Delay8/1 -> Bus Creator/9  "TCP Rotational Speed Command (rpm)"
  [omega_AuxTCP_rpm_Get] -> Unit Delay11/1
  [omega_AuxTCP_rpm_Set] -> Unit Delay10/1
  Unit Delay10/1 -> Bus Creator/11  "AuxTCP Rotational Speed Command (rpm)"
  Unit Delay11/1 -> Bus Creator/12  "AuxTCP Rotational Speed (rpm)"
  Kelvin to °C/1(Temp. (°C)) -> Bus Creator/1  "Stack Inlet Temperature: TSens_CLSti 6812 (°C)"
  Kelvin to °C1/1(Temp. (°C)) -> Bus Creator/2  "Stack Outlet Temperature: TSens_CLSto 6820 (°C)"
  Kelvin to °C2/1(Temp. (°C)) -> Bus Creator/6  "TCV Inlet Temperature: TSens_TCVi 6801 (°C)"
  Pascal to Bar(a)/1(Press. Bar(a)) -> Bus Creator/3  "TCP Inlet Pressure: pSens_TCPi 6811 (Bar)"
  Pascal to Bar(a)1/1(Press. Bar(a)) -> Bus Creator/4  "Stack Inlet Pressure: pSens_CLSti 6812 (Bar)"
  Pascal to Bar(a)2/1(Press. Bar(a)) -> Bus Creator/5  "TCV Inlet Pressure: pSens_TCVi 6801 (Bar)"
  Rate Transition/1 -> [pos_TCV_per_Set], Transfer Fcn/1
  Transfer Fcn/1 -> Rate Limiter/1
  Rate Transition1/1 -> Transfer Fcn1/1, [omega_AuxTCP_rpm_Set]
  Transfer Fcn1/1 -> Rate Limiter1/1
  Transfer Fcn2/1 -> Rate Limiter2/1
  Rate Transition2/1 -> Transfer Fcn2/1, [omega_TCP_rpm_Set]
  Unit Delay13/1 -> Bus Creator/15  "Cold Circuit Coolant Massflow (kg/s)"
  Unit Delay12/1 -> Bus Creator/14  "Hot Circuit Coolant Massflow (kg/s)"
  [mDot_Overall_kgs] -> Unit Delay14/1
  Unit Delay14/1 -> Bus Creator/13  "Overall Coolant Massflow (kg/s)"
  [mDot_Cold_kgs] -> Unit Delay13/1
  [mDot_Hot_kgs] -> Unit Delay12/1
  [omega_AuxTCP_rpm_Get] -> Pumps RPM/4
  [omega_TCP_rpm_Get] -> Pumps RPM/2
  [omega_AuxTCP_rpm_Set] -> Pumps RPM/3
  PS-Simulink Converter26/1 -> Goto27/1  "Bypass Mass Flow (kg/s)"
  PS-Simulink Converter27/1 -> Terminator5/1
  [mDot_Bypass_kgs] -> Massflow/4
  [mDot_Bypass_kgs] -> Unit Delay15/1
  Unit Delay15/1 -> Bus Creator/16  "Bypass Coolant Massflow (kg/s)"
  PS-Simulink Converter29/1 -> Terminator6/1
  PS-Simulink Converter28/1 -> [mDot_AuxTCP_kgs]  "AuxTCP Mass Flow (kg/s)"
  [mDot_AuxTCP_kgs] -> Massflow/5
  Current to Heat/1 -> Simulink-PS Converter3/1
  Stack Current (A)/1 -> Rate Transition3/1
  Rate Transition3/1 -> Current to Heat/1, [I_SFC_A]
  [I_SFC_A] -> Unit Delay16/1
  Unit Delay16/1 -> Bus Creator/17  "Stack Current: I_A_StN (A)"
  Constant/1 -> Simulink-PS Converter4/1
  Constant1/1 -> Aircraft Duct/1(V_air)
  TCV_in Temperature (K)/1 -> Low-Pass Filter (Discrete or Continuous)/1
  Rate Transition4/1 -> Aircraft Duct/2(T_air)
  Low-Pass Filter (Discrete or Continuous)/1 -> Rate Transition4/1
  connections:
  Fuel Cell Coolant Channels/LConn2 -- Solver Configuration/RConn1 -- Heat Flow Rate Sensor1/RConn2 -- PS100-P02Stack Thermal Mass/LConn1
  Ideal Angular Velocity Source/LConn1 -- Ideal Rotational Motion Sensor/LConn1 -- Ideal Torque Sensor/LConn1
  Ideal Rotational Motion Sensor/RConn1 -- TCP (6812)/RConn2 -- Mechanical Rotational Reference1/LConn1
  Pressure & Temperature Sensor (TL)2/LConn1 -- Glysantin G20 (Ethylenglykol/Water)/RConn1 -- Pipe (TL)2/LConn1 -- Mass & Energy Flow Rate Sensor (TL)/RConn1
  Pressure & Temperature Sensor (TL)5/LConn1 -- Mass & Energy Flow Rate Sensor (TL)1/RConn1 -- TCV (VL6810)/RConn2
  Radiator/LConn2 -- Coolant Tank/RConn1 -- Pressure & Temperature Sensor (TL)6/LConn1 -- Mass & Energy Flow Rate Sensor (TL)4/LConn1
  Ideal Torque Sensor/RConn2 -- PS-Simulink Converter6/LConn1 -- PS Product/LConn1
  Ideal Rotational Motion Sensor/RConn2 -- PS Product/LConn2 -- PS-Simulink Converter 1/LConn1
  Ideal Angular Velocity Source1/LConn1 -- Ideal Rotational Motion Sensor1/LConn1 -- Ideal Torque Sensor1/LConn1
  Ideal Torque Sensor1/RConn2 -- PS-Simulink Converter25/LConn1 -- PS Product1/LConn1
  Mechanical Rotational Reference2/LConn1 -- Aux TCP/RConn2 -- Ideal Rotational Motion Sensor1/RConn1
  Ideal Rotational Motion Sensor1/RConn2 -- PS Product1/LConn2 -- PS-Simulink Converter 2/LConn1
  Pressure & Temperature Sensor (TL)1/LConn1 -- Fuel Cell Coolant Channels/LConn1 -- Pipe (TL)2/RConn1
  Fuel Cell Coolant Channels/RConn1 -- T-Junction (TL)/LConn1 -- Pressure & Temperature Sensor (TL)4/LConn1
  Mass & Energy Flow Rate Sensor (TL)1/LConn1 -- Aux TCP/LConn2 -- Mass & Energy Flow Rate Sensor (TL)3/RConn1
  Pressure & Temperature Sensor (TL)3/LConn1 -- TCP (6812)/LConn1 -- Pipe (TL)1/RConn1
  Pipe (TL)3/RConn1 -- Radiator/LConn1 -- Gate Valve (TL)/LConn1
  Heat Flow Rate Sensor1/RConn1 -- PS-Simulink Converter12/LConn1
  Mechanical Rotational Reference3/LConn1 -- Ideal Angular Velocity Source/RConn2
  PS-Simulink Converter11/LConn1 -- Ideal Rotational Motion Sensor/RConn3
  Simulink-PS Converter/RConn1 -- TCV (VL6810)/RConn1
  Simulink-PS Converter3/RConn1 -- Controlled Heat Flow Rate Source/RConn1
  Controlled Heat Flow Rate Source/LConn1 -- Heat Flow Rate Sensor1/LConn1
  Thermal Reference/LConn1 -- Controlled Heat Flow Rate Source/RConn2
  TCP (6812)/RConn1 -- Ideal Torque Sensor/RConn1
  Simulink-PS Converter2/RConn1 -- Ideal Angular Velocity Source/RConn1
  Absolute Reference (TL)1/LConn1 -- Pressure & Temperature Sensor (TL)1/RConn1
  PS-Simulink Converter7/LConn1 -- Pressure & Temperature Sensor (TL)1/RConn3
  Pressure & Temperature Sensor (TL)1/RConn2 -- PS-Simulink Converter/LConn1
  Absolute Reference (TL)2/LConn1 -- Pressure & Temperature Sensor (TL)2/RConn1
  Absolute Reference (TL)3/LConn1 -- Pressure & Temperature Sensor (TL)3/RConn1
  Pressure & Temperature Sensor (TL)4/RConn1 -- Absolute Reference (TL)4/LConn1
  Pressure & Temperature Sensor (TL)4/RConn2 -- PS-Simulink Converter9/LConn1
  PS-Simulink Converter10/LConn1 -- Pressure & Temperature Sensor (TL)4/RConn3
  Pressure & Temperature Sensor (TL)3/RConn2 -- PS-Simulink Converter4/LConn1
  Pressure & Temperature Sensor (TL)3/RConn3 -- PS-Simulink Converter5/LConn1
  Pressure & Temperature Sensor (TL)2/RConn3 -- PS-Simulink Converter8/LConn1
  Pressure & Temperature Sensor (TL)2/RConn2 -- PS-Simulink Converter1/LConn1
  Mass & Energy Flow Rate Sensor (TL)/RConn3 -- PS-Simulink Converter3/LConn1
  Mass & Energy Flow Rate Sensor (TL)/RConn2 -- PS-Simulink Converter13/LConn1
  Mass & Energy Flow Rate Sensor (TL)1/RConn2 -- PS-Simulink Converter14/LConn1
  Mass & Energy Flow Rate Sensor (TL)1/RConn3 -- PS-Simulink Converter15/LConn1
  Pressure & Temperature Sensor (TL)5/RConn3 -- PS-Simulink Converter17/LConn1
  Absolute Reference (TL)5/LConn1 -- Pressure & Temperature Sensor (TL)5/RConn1
  Pressure & Temperature Sensor (TL)5/RConn2 -- PS-Simulink Converter16/LConn1
  Pressure & Temperature Sensor (TL)6/RConn2 -- PS-Simulink Converter21/LConn1
  Pressure & Temperature Sensor (TL)6/RConn1 -- Absolute Reference (TL)6/LConn1
  Mass & Energy Flow Rate Sensor (TL)2/RConn2 -- PS-Simulink Converter22/LConn1
  Mass & Energy Flow Rate Sensor (TL)2/RConn3 -- PS-Simulink Converter23/LConn1
  PS-Simulink Converter24/LConn1 -- PS Product/RConn1
  PS-Simulink Converter19/LConn1 -- PS Product1/RConn1
  PS-Simulink Converter18/LConn1 -- Ideal Rotational Motion Sensor1/RConn3
  Aux TCP/RConn1 -- Ideal Torque Sensor1/RConn1
  Mechanical Rotational Reference4/LConn1 -- Ideal Angular Velocity Source1/RConn2
  Simulink-PS Converter1/RConn1 -- Ideal Angular Velocity Source1/RConn1
  TCP (6812)/LConn2 -- Mass & Energy Flow Rate Sensor (TL)/LConn1
  Perfect Insulator/LConn1 -- Pipe (TL)2/LConn2
  Perfect Insulator1/LConn1 -- Pipe (TL)3/LConn2
  Perfect Insulator2/LConn1 -- Pipe (TL)4/LConn2
  Pipe (TL)4/LConn1 -- Mass & Energy Flow Rate Sensor (TL)2/RConn1
  Pipe (TL)4/RConn1 -- TCV (VL6810)/RConn3
  Mass & Energy Flow Rate Sensor (TL)4/RConn1 -- Aux TCP/LConn1
  PS-Simulink Converter28/LConn1 -- Mass & Energy Flow Rate Sensor (TL)4/RConn2
  PS-Simulink Converter29/LConn1 -- Mass & Energy Flow Rate Sensor (TL)4/RConn3
  Pressure & Temperature Sensor (TL)6/RConn3 -- PS-Simulink Converter20/LConn1
  Simulink-PS Converter4/RConn1 -- Gate Valve (TL)/LConn2
  Mass & Energy Flow Rate Sensor (TL)3/LConn1 -- Gate Valve (TL)/RConn1
  PS-Simulink Converter27/LConn1 -- Mass & Energy Flow Rate Sensor (TL)3/RConn3
  PS-Simulink Converter26/LConn1 -- Mass & Energy Flow Rate Sensor (TL)3/RConn2
  Radiator/RConn3 -- Aircraft Duct/RConn3
  Radiator/RConn2 -- Aircraft Duct/RConn2
  Radiator/RConn1 -- Aircraft Duct/RConn1
  T-Junction (TL)/RConn2 -- Mass & Energy Flow Rate Sensor (TL)2/LConn1
  Pipe (TL)3/LConn1 -- T-Junction (TL)/RConn1
  TCV (VL6810)/LConn1 -- Flow Resistance (TL)/LConn1
  Pipe (TL)1/LConn1 -- Flow Resistance (TL)/RConn1
  Perfect Insulator3/LConn1 -- Pipe (TL)1/LConn2

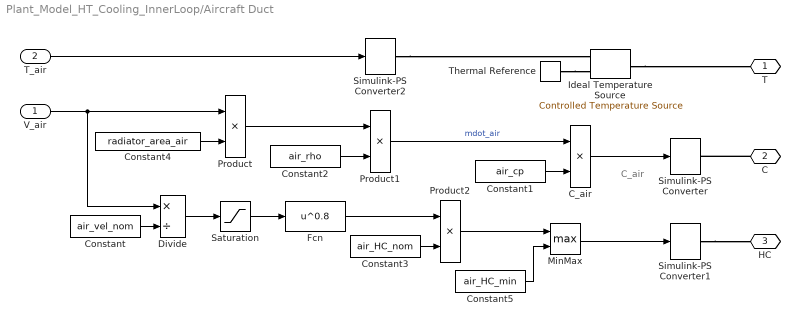
== system Plant_Model_HT_Cooling_InnerLoop/Aircraft Duct ==
  note: C_air
  V_air : Inport
  T_air : Inport  Port=2
  C_air : Product
  Constant : Constant  Value=air_vel_nom
  Constant1 : Constant  Value=air_cp
  Constant2 : Constant  Value=air_rho
  Constant3 : Constant  Value=air_HC_nom
  Constant4 : Constant  Value=radiator_area_air
  Constant5 : Constant  Value=air_HC_min
  Divide : Product  Inputs=*/
  Fcn : Fcn  Expr=u^0.8
  Ideal Temperature Source : fl_lib/Thermal/Thermal Sources/Controlled Temperature Source
  MinMax : MinMax  Function=max  Inputs=2
  Product : Product
  Product1 : Product
  Product2 : Product
  Saturation : Saturate  UpperLimit=inf  LowerLimit=0
  Simulink-PS Converter : nesl_utility/Simulink-PS Converter  PhysicalDomain=network_engine_domain  SubClassName=ps_input  LeftPortType=input  RightPortType=output  PseudoPeriodic=off  Frequencies=[]  NoiseDistribution=none  NoiseParameters=[]  Unit=W/K  AffineConversion=off  FilteringAndDerivatives=zero  SimscapeFilterOrder=1  InputFilterTimeConstant=1  UdotUserProvided=1
  Simulink-PS Converter1 : nesl_utility/Simulink-PS Converter  PhysicalDomain=network_engine_domain  SubClassName=ps_input  LeftPortType=input  RightPortType=output  PseudoPeriodic=off  Frequencies=[]  NoiseDistribution=none  NoiseParameters=[]  Unit=W/(m^2*K)  AffineConversion=off  FilteringAndDerivatives=zero  SimscapeFilterOrder=1  InputFilterTimeConstant=1  UdotUserProvided=1
  Simulink-PS Converter2 : nesl_utility/Simulink-PS Converter  PhysicalDomain=network_engine_domain  SubClassName=ps_input  LeftPortType=input  RightPortType=output  PseudoPeriodic=off  Frequencies=[]  NoiseDistribution=none  NoiseParameters=[]  Unit=K  AffineConversion=on  FilteringAndDerivatives=zero  SimscapeFilterOrder=1  InputFilterTimeConstant=1  UdotUserProvided=1
  Thermal Reference : fl_lib/Thermal/Thermal Elements/Thermal Reference
  T : PMIOPort  Side=Right
  C : PMIOPort  Port=2  Side=Right
  HC : PMIOPort  Port=3  Side=Right
  wires:
  Saturation/1 -> Fcn/1
  Product1/1 -> C_air/1  "mdot_air"
  Constant4/1 -> Product/2
  Constant2/1 -> Product1/2
  Product/1 -> Product1/1
  C_air/1 -> Simulink-PS Converter/1
  Constant1/1 -> C_air/2
  T_air/1 -> Simulink-PS Converter2/1
  MinMax/1 -> Simulink-PS Converter1/1
  Constant5/1 -> MinMax/2
  Product2/1 -> MinMax/1
  Fcn/1 -> Product2/1
  Divide/1 -> Saturation/1
  Constant3/1 -> Product2/2
  Constant/1 -> Divide/2
  V_air/1 -> Divide/1, Product/1
  connections:
  Ideal Temperature Source/LConn1 -- T/RConn1
  Simulink-PS Converter2/RConn1 -- Ideal Temperature Source/RConn1
  Thermal Reference/LConn1 -- Ideal Temperature Source/RConn2
  Simulink-PS Converter1/RConn1 -- HC/RConn1
  C/RConn1 -- Simulink-PS Converter/RConn1

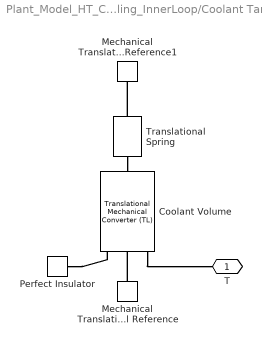
== system Plant_Model_HT_Cooling_InnerLoop/Coolant Tank ==
  Coolant Volume : fl_lib/Thermal Liquid/Elements/Translational Mechanical Converter (TL)  mech_orientation=foundation.enum.MechOrientationTranslational.Positive  displacement_spec=foundation.enum.DisplacementSpec.Calculate  x0=x_init m  interface_area=A m^2  dead_volume=A * 0.001 m^3  environment_spec=foundation.enum.pressure_spec.specified  environment_pressure=coolant_initial_pressure MPa  dynamic_compressibility=simscape.enum.onoff.off  p0=env_p MPa  T0=coolant_initial_temperature K
      settings: InternalSimscapePortConfiguration="{\"Bottom\":[],\"Left\":[{\"id\":\"A\",\"label\":\"A\",\"type\":\"foundation.thermal_liquid.thermal_liquid\"},{\"id\":\"C\",\"label\":\"C\",\"type\":\"foundation.mechanical.translational.translational\"},{\"id\":\"H\",\"label\":\"H\",\"type\":\"foundation.thermal.thermal\"}],\"Right\":[{\"id\":\"R\",\"label\":\"R\",\"type\":\"foundation.mechanical.translational.translational\"}],\"Top\":[]}"
  Mechanical Translational Reference : fl_lib/Mechanical/Translational Elements/Mechanical Translational Reference
  Mechanical Translational Reference1 : fl_lib/Mechanical/Translational Elements/Mechanical Translational Reference
  Perfect Insulator : fl_lib/Thermal/Thermal Elements/Perfect Insulator  T_specify=off  T_priority=None  T=0 K  T_nominal_specify=off  T_nominal_unit=K  T_nominal_value=1
  Translational Spring : fl_lib/Mechanical/Translational Elements/Translational Spring  spr_rate=1e6 N/m  v_specify=off  v_priority=None  v=0 m/s  v_nominal_specify=off  v_nominal_unit=m/s  v_nominal_value=1  f_specify=off  f_priority=None  f=0 N  f_nominal_specify=off  f_nominal_unit=N  f_nominal_value=1  x_specify=off  x_priority=High  x=x_init m  x_nominal_specify=on  x_nominal_unit=m  x_nominal_value=x_init
  T : PMIOPort  Side=Right
  connections:
  Translational Spring/LConn1 -- Mechanical Translational Reference1/LConn1
  Translational Spring/RConn1 -- Coolant Volume/RConn1
  Perfect Insulator/LConn1 -- Coolant Volume/LConn3
  Mechanical Translational Reference/LConn1 -- Coolant Volume/LConn2
  Coolant Volume/LConn1 -- T/RConn1

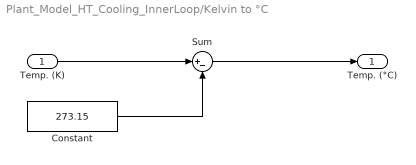
== system Plant_Model_HT_Cooling_InnerLoop/Kelvin to °C ==
  Temp. (K) : Inport
  Constant : Constant  Value=273.15
  Sum : Sum  Inputs=|+-
  Temp. (°C) : Outport
  wires:
  Temp. (K)/1 -> Sum/1
  Sum/1 -> Temp. (°C)/1
  Constant/1 -> Sum/2

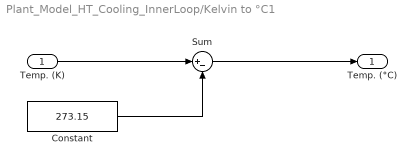
== system Plant_Model_HT_Cooling_InnerLoop/Kelvin to °C1 ==
  Temp. (K) : Inport
  Constant : Constant  Value=273.15
  Sum : Sum  Inputs=|+-
  Temp. (°C) : Outport
  wires:
  Temp. (K)/1 -> Sum/1
  Sum/1 -> Temp. (°C)/1
  Constant/1 -> Sum/2

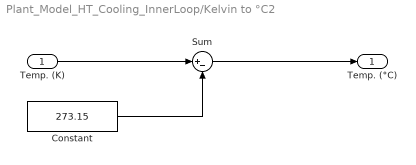
== system Plant_Model_HT_Cooling_InnerLoop/Kelvin to °C2 ==
  Temp. (K) : Inport
  Constant : Constant  Value=273.15
  Sum : Sum  Inputs=|+-
  Temp. (°C) : Outport
  wires:
  Temp. (K)/1 -> Sum/1
  Sum/1 -> Temp. (°C)/1
  Constant/1 -> Sum/2

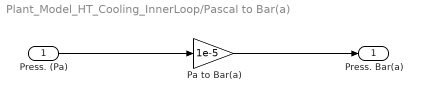
== system Plant_Model_HT_Cooling_InnerLoop/Pascal to Bar(a) ==
  Press. (Pa) : Inport
  Pa to Bar(a) : Gain  Gain=1e-5
  Press. Bar(a) : Outport
  wires:
  Press. (Pa)/1 -> Pa to Bar(a)/1
  Pa to Bar(a)/1 -> Press. Bar(a)/1

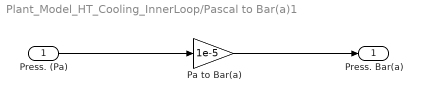
== system Plant_Model_HT_Cooling_InnerLoop/Pascal to Bar(a)1 ==
  Press. (Pa) : Inport
  Pa to Bar(a) : Gain  Gain=1e-5
  Press. Bar(a) : Outport
  wires:
  Press. (Pa)/1 -> Pa to Bar(a)/1
  Pa to Bar(a)/1 -> Press. Bar(a)/1

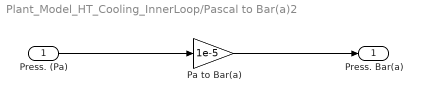
== system Plant_Model_HT_Cooling_InnerLoop/Pascal to Bar(a)2 ==
  Press. (Pa) : Inport
  Pa to Bar(a) : Gain  Gain=1e-5
  Press. Bar(a) : Outport
  wires:
  Press. (Pa)/1 -> Pa to Bar(a)/1
  Pa to Bar(a)/1 -> Press. Bar(a)/1

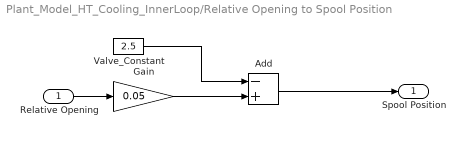
== system Plant_Model_HT_Cooling_InnerLoop/Relative Opening to Spool Position ==
  Relative Opening : Inport
  Add : Sum  Inputs=-+
  Gain : Gain  Gain=0.05
  Valve_Constant : Constant  Value=2.5
  Spool Position : Outport
  wires:
  Add/1 -> Spool Position/1
  Valve_Constant/1 -> Add/1
  Relative Opening/1 -> Gain/1
  Gain/1 -> Add/2
